simulink model "sampleModel2051"  (R2023a)
settings: Solver=VariableStepAuto  StartTime=0.0  StopTime=10.0  RelTol=1e-3
libraries: simulink x5, hdlsllib x4
settings Model: Creator=user1  LastModifiedBy=user1

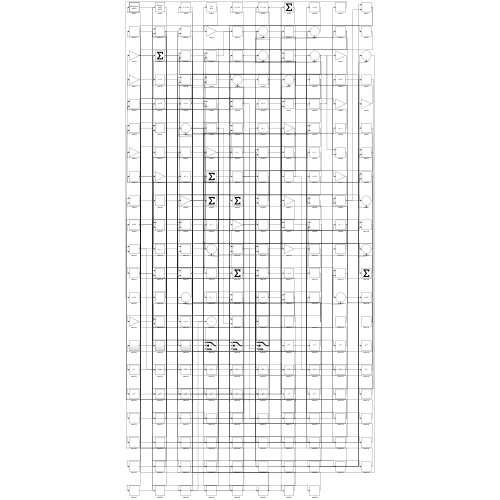
[thumbnail: Simulink's stored preview of the top-level diagram]
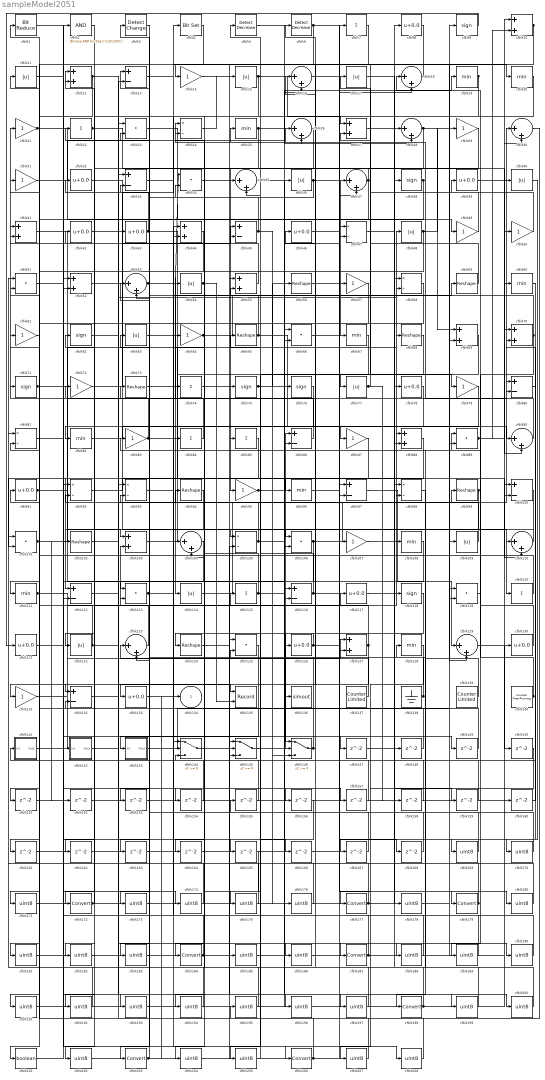
== system sampleModel2051 ==
  cfblk1 : hdlsllib/Logic and Bit Operations/Bit Reduce  mode=AND
  cfblk{10,12,27,41,44,52,55,69..70,88,103,127} (12 alike) : Sum
  cfblk{13,33,45,80,86,97,100,112,116,132} (10 alike) : Sum  Inputs=+-
  cfblk{23,34,51,66,89,101,106,113,119,125} (10 alike) : DotProduct  OutDataTypeStr=Inherit: Inherit via internal rule
  cfblk{56,59,65,68,73,94,99,102,124} (9 alike) : Reshape
  cfblk{16,18,26,28,30,35,37,53,90,104,110,123,129} (13 alike) : Sum  Inputs=|++
  cfblk{24,47,58,81,92..93,98,105} (8 alike) : Product  Inputs=*/  RndMeth=Zero  SaturateOnIntegerOverflow=on
  cfblk{14,21,29,31,49..50,57,61,64,72,79,83,87,95,107,131} (16 alike) : Gain
  cfblk{19..20,25,60,67,82,96,108,111,128} (10 alike) : MinMax
  cfblk{11,15,17,36,40,48,54,63,77,109,114,122} (12 alike) : Abs  SaturateOnIntegerOverflow=off
  cfblk{7,22,74,84..85,115,120} (7 alike) : Sum  Inputs=+
  cfblk{8,32,39,42..43,46,78,91,117,121,126,130,133} (13 alike) : Bias  Bias=0.0  SaturateOnIntegerOverflow=off
  cfblk{9,38,62,71,75..76,118} (7 alike) : Signum
  cfblk135 : Record  FileSettingsInternal="{\"entries\":[{\"content\":{\"excelSettings\":{\"content\":{},\"type\":\"Streamout.ExcelSettings\"}},\"type\":\"Streamout.FileSettingStorage\",\"uuid\":\"\"}],\"packageUris\":[\"http:\\/\\/schema.mathworks.com\\/mf0\\/streamout_blocks\\/R2020a\"],\"version\":\"1.0\"}"  Layout=[1 1]  SignalsInternal="{\"entries\":[{\"content\":{\"signals\":[{\"content\":{\"blockPath\":[],\"dimensions\":[1],\"domain\":\"\",\"lineColor\":\"#a2142f\",\"plots\":[1],\"port\":1,\"signalID\":6285,\"signalName\":\"XY Graph:1\"},\"type\":\"RecordBlkView.Signal\",\"uuid\":\"\"},{\"content\":{\"blockPath\":[],\"dimensions\":[1],\"domain\":\"\",\"lineColor\":\"#139fff\",\"plots\":[1],\"port\":2,\"signalID\":6288,\"signalName\":\"XY Graph:2\"},\"type\":\"RecordBlkView.Signal\",\"uuid\":\"\"}]},\"type\":\"RecordBlkView.InputSignals\",\"uuid\":\"\"}],\"packageUris\":[\"http:\\/\\/schema.mathworks.com\\/mf0\\/streamout_blocks\\/R2020a\"],\"version\":\"1.0\"}"  VisualizationBindings="{\"xyplotplugin\":{\"info\":[{\"series\":[{\"bindingParametersList\":[{\"parameter\":\"X-Axis\",\"signalID\":6285,\"signalName\":\"XY Graph:1\"},{\"parameter\":\"Y-Axis\",\"signalID\":6288,\"signalName\":\"XY Graph:2\"}],\"seriesID\":30765}],\"subplotID\":1}]}}"  CompatibilityTag=XY  st=-1
  cfblk136 : ToWorkspace  VariableName=simout  SaveFormat=Timeseries  SampleTime=-1
  cfblk137 : hdlsllib/Sources/Counter Limited  uplimit=7  tsamp=-1
  cfblk138 : Ground
  cfblk139 : hdlsllib/Sources/Counter Limited  uplimit=7  tsamp=-1
  cfblk140 : hdlsllib/Sources/Counter Free-Running  NumBits=16  tsamp=-1
  cfblk141 : Subsystem
      settings: LibrarySourceBlock=|
      | hdlsllib/Ports &
      | Subsystems/Subsystem
  cfblk142 : Subsystem
      settings: LibrarySourceBlock=|
      | hdlsllib/Ports &
      | Subsystems/Subsystem
  cfblk143 : Subsystem
      settings: LibrarySourceBlock=|
      | hdlsllib/Ports &
      | Subsystems/Subsystem
  cfblk144 : Switch  SaturateOnIntegerOverflow=off  InputSameDT=off
  cfblk145 : Switch  SaturateOnIntegerOverflow=off  InputSameDT=off
  cfblk146 : Switch  SaturateOnIntegerOverflow=off  InputSameDT=off
  cfblk{147..168} (22 alike) : Delay  SampleTime=1
  cfblk{169..171,173..176,178,180..183,185..186,188..197,199..200,202,204..205,207..208} (31 alike) : DataTypeConversion  OutDataTypeStr=uint8  SaturateOnIntegerOverflow=off  RndMeth=Floor
  cfblk{172,177,179,184,187,198,203,206} (8 alike) : DataTypeConversion  SaturateOnIntegerOverflow=off  RndMeth=Floor
  cfblk2 : simulink/Logic and Bit Operations/Bitwise Operator  logicop=AND  UseBitMask=on  BitMask=bin2dec('11011001')  BitMaskRealWorld=Stored Integer
      settings: LibrarySourceBlock=|
      | hdlsllib/Logic and Bit
      | Operations/Bitwise
      | Operator
  cfblk201 : DataTypeConversion  OutDataTypeStr=boolean  SaturateOnIntegerOverflow=off  RndMeth=Floor
  cfblk3 : simulink/Logic and Bit Operations/Detect Change  vinit=0  OutDataTypeStr=boolean
      settings: LibrarySourceBlock=|
      | hdlsllib/Logic and Bit
      | Operations/Detect
      | Change
  cfblk4 : simulink/Logic and Bit Operations/Bit Set  iBit=0
      settings: LibrarySourceBlock=|
      | hdlsllib/Logic and Bit
      | Operations/Bit Set
  cfblk5 : simulink/Logic and Bit Operations/Detect Decrease  vinit=0.0  OutDataTypeStr=boolean
      settings: LibrarySourceBlock=|
      | hdlsllib/Logic and Bit
      | Operations/Detect
      | Decrease
  cfblk6 : simulink/Logic and Bit Operations/Detect Decrease  vinit=0.0  OutDataTypeStr=boolean
      settings: LibrarySourceBlock=|
      | hdlsllib/Logic and Bit
      | Operations/Detect
      | Decrease
  cfblk134 : Outport  VectorParamsAs1DForOutWhenUnconnected=off
  wires:
  cfblk48/1 -> cfblk114/1, cfblk29/1
  cfblk41/1 -> cfblk103/1
  cfblk141/1(Out1) -> cfblk127/1
  cfblk145/1 -> cfblk86/1
  cfblk18/1 -> cfblk14/1
  cfblk66/1 -> cfblk37/1
  cfblk64/1 -> cfblk38/1, cfblk204/1
  cfblk55/1 -> cfblk42/1
  cfblk88/1 -> cfblk112/1
  cfblk78/1 -> cfblk172/1
  cfblk3/1 -> cfblk143/1(In1)
  cfblk84/1 -> cfblk21/1
  cfblk90/1 -> cfblk26/1
  cfblk9/1 -> cfblk121/1
  cfblk26/1 -> cfblk95/1
  cfblk60/1 -> cfblk141/1(In1)
  cfblk72/1 -> cfblk45/1
  cfblk117/1 -> cfblk48/1
  cfblk10/1 -> cfblk77/1, cfblk69/2
  cfblk146/1 -> cfblk46/1, cfblk92/2
  cfblk23/1 -> cfblk49/1
  cfblk111/1 -> cfblk117/1, cfblk145/2
  cfblk15/1 -> cfblk27/1, cfblk44/2
  cfblk103/1 -> cfblk68/1
  cfblk125/1 -> cfblk203/1
  cfblk32/1 -> cfblk120/1
  cfblk140/1 -> cfblk18/1, cfblk83/1
  cfblk118/1 -> cfblk146/1
  cfblk112/1 -> cfblk33/1
  cfblk92/1 -> cfblk96/1
  cfblk21/1 -> cfblk55/1, cfblk166/1
  cfblk47/1 -> cfblk28/1
  cfblk65/1 -> cfblk87/1, cfblk23/2
  cfblk8/1 -> cfblk136/1
  cfblk59/1 -> cfblk27/2
  cfblk126/1 -> cfblk118/1, cfblk124/1
  cfblk123/1 -> cfblk103/2
  cfblk143/1(Out1) -> cfblk9/1
  cfblk113/1 -> cfblk59/1, cfblk173/1
  cfblk114/1 -> cfblk30/1
  cfblk25/1 -> cfblk28/2, cfblk82/1
  cfblk105/1 -> cfblk13/1, cfblk146/3, cfblk197/1
  cfblk53/1 -> cfblk34/1, cfblk156/1, cfblk157/1
  cfblk70/1 -> cfblk22/1, cfblk189/1
  cfblk49/1 -> cfblk24/1
  cfblk97/1 -> cfblk129/1
  cfblk69/1 -> cfblk86/2
  cfblk35/1 -> cfblk76/1
  cfblk37/1 -> cfblk35/1, cfblk201/1
  cfblk137/1 -> cfblk123/1
  cfblk115/1 -> cfblk41/1, cfblk199/1
  cfblk100/1 -> cfblk184/1
  cfblk128/1 -> cfblk177/1
  cfblk91/1 -> cfblk8/1, cfblk154/1
  cfblk77/1 -> cfblk17/1, cfblk158/1
  cfblk13/1 -> cfblk20/1
  cfblk31/1 -> cfblk19/1
  cfblk87/1 -> cfblk101/2
  cfblk127/1 -> cfblk12/1, cfblk151/1, cfblk163/1
  cfblk46/1 -> cfblk97/1
  cfblk24/1 -> cfblk15/1
  cfblk138/1 -> cfblk73/1, cfblk127/2, cfblk41/2
  cfblk144/1 -> cfblk187/1
  cfblk45/1 -> cfblk3/1, cfblk176/1
  cfblk89/1 -> cfblk10/1, cfblk10/2
  cfblk139/1 -> cfblk88/1
  cfblk28/1 -> cfblk123/2, cfblk88/2, cfblk69/1
  cfblk116/1 -> cfblk7/1, cfblk5/1
  cfblk73/1 -> cfblk90/1
  cfblk109/1 -> cfblk94/1
  cfblk43/1 -> cfblk145/1, cfblk32/1
  cfblk11/1 -> cfblk142/1(In1)
  cfblk36/1 -> cfblk34/2, cfblk89/2
  cfblk58/1 -> cfblk75/1
  cfblk50/1 -> cfblk25/1
  cfblk110/1 -> cfblk105/1
  cfblk12/1 -> cfblk161/1, cfblk162/1, cfblk200/1
  cfblk14/1 -> cfblk97/2
  cfblk101/1 -> cfblk80/1, cfblk152/1
  cfblk29/1 -> cfblk133/1
  cfblk104/1 -> cfblk112/2
  cfblk122/1 -> cfblk99/1, cfblk11/1
  cfblk120/1 -> cfblk91/1
  cfblk98/1 -> cfblk198/1
  cfblk54/1 -> cfblk104/1, cfblk135/2
  cfblk95/1 -> cfblk47/1, cfblk149/1
  cfblk96/1 -> cfblk18/2
  cfblk75/1 -> cfblk110/1, cfblk56/1, cfblk190/1
  cfblk7/1 -> cfblk45/2
  cfblk52/1 -> cfblk4/1
  cfblk39/1 -> cfblk90/2
  cfblk5/1 -> cfblk26/2
  cfblk19/1 -> cfblk113/1, cfblk104/2
  cfblk83/1 -> cfblk110/2, cfblk80/2, cfblk31/1, cfblk106/2
  cfblk68/1 -> cfblk106/1
  cfblk71/1 -> cfblk52/2, cfblk126/1
  cfblk44/1 -> cfblk111/1
  cfblk63/1 -> cfblk79/1
  cfblk16/1 -> cfblk179/1
  cfblk99/1 -> cfblk39/1, cfblk192/1
  cfblk22/1 -> cfblk129/2, cfblk60/1
  cfblk93/1 -> cfblk206/1
  cfblk82/1 -> cfblk84/1
  cfblk86/1 -> cfblk54/1
  cfblk133/1 -> cfblk55/2
  cfblk106/1 -> cfblk70/1, cfblk164/1
  cfblk62/1 -> cfblk135/1
  cfblk131/1 -> cfblk43/1
  cfblk76/1 -> cfblk132/1
  cfblk33/1 -> cfblk85/1
  cfblk79/1 -> cfblk146/2
  cfblk142/1(Out1) -> cfblk115/1
  cfblk132/1 -> cfblk58/2
  cfblk6/1 -> cfblk107/1, cfblk145/3
  cfblk130/1 -> cfblk89/1
  cfblk57/1 -> cfblk131/1
  cfblk38/1 -> cfblk102/1, cfblk171/1
  cfblk20/1 -> cfblk122/1
  cfblk121/1 -> cfblk147/1
  cfblk27/1 -> cfblk148/1
  cfblk148/1 -> cfblk52/1
  cfblk149/1 -> cfblk1/1
  cfblk129/1 -> cfblk150/1
  cfblk151/1 -> cfblk30/2
  cfblk152/1 -> cfblk13/2
  cfblk85/1 -> cfblk153/1
  cfblk153/1 -> cfblk33/2
  cfblk154/1 -> cfblk53/1
  cfblk155/1 -> cfblk132/2
  cfblk157/1 -> cfblk12/2
  cfblk158/1 -> cfblk35/2
  cfblk17/1 -> cfblk159/1
  cfblk159/1 -> cfblk24/2
  cfblk160/1 -> cfblk70/2
  cfblk161/1 -> cfblk105/2
  cfblk162/1 -> cfblk44/1
  cfblk163/1 -> cfblk37/2
  cfblk164/1 -> cfblk47/2
  cfblk42/1 -> cfblk165/1
  cfblk166/1 -> cfblk116/2
  cfblk40/1 -> cfblk167/1
  cfblk167/1 -> cfblk66/1
  cfblk56/1 -> cfblk168/1
  cfblk168/1 -> cfblk58/1
  cfblk119/1 -> cfblk169/1
  cfblk169/1 -> cfblk63/1
  cfblk80/1 -> cfblk170/1
  cfblk170/1 -> cfblk119/1
  cfblk171/1 -> cfblk119/2
  cfblk172/1 -> cfblk72/1, cfblk62/1
  cfblk173/1 -> cfblk78/1
  cfblk51/1 -> cfblk174/1
  cfblk174/1 -> cfblk23/1
  cfblk156/1 -> cfblk175/1
  cfblk175/1 -> cfblk51/1
  cfblk176/1 -> cfblk51/2
  cfblk177/1 -> cfblk64/1, cfblk101/1
  cfblk107/1 -> cfblk178/1
  cfblk178/1 -> cfblk128/1
  cfblk179/1 -> cfblk65/1, cfblk116/1
  cfblk147/1 -> cfblk180/1
  cfblk180/1 -> cfblk16/1
  cfblk4/1 -> cfblk181/1
  cfblk181/1 -> cfblk16/2
  cfblk108/1 -> cfblk182/1
  cfblk182/1 -> cfblk57/1
  cfblk94/1 -> cfblk183/1
  cfblk183/1 -> cfblk108/1
  cfblk184/1 -> cfblk92/1, cfblk36/1
  cfblk124/1 -> cfblk185/1
  cfblk185/1 -> cfblk100/1
  cfblk102/1 -> cfblk186/1
  cfblk186/1 -> cfblk100/2
  cfblk187/1 -> cfblk155/1, cfblk109/1
  cfblk34/1 -> cfblk188/1
  cfblk188/1 -> cfblk144/1
  cfblk189/1 -> cfblk144/2
  cfblk190/1 -> cfblk144/3
  cfblk61/1 -> cfblk191/1
  cfblk191/1 -> cfblk50/1
  cfblk192/1 -> cfblk61/1
  cfblk81/1 -> cfblk193/1
  cfblk193/1 -> cfblk66/2
  cfblk165/1 -> cfblk194/1
  cfblk194/1 -> cfblk81/1
  cfblk30/1 -> cfblk195/1
  cfblk195/1 -> cfblk81/2
  cfblk74/1 -> cfblk196/1
  cfblk196/1 -> cfblk40/1
  cfblk197/1 -> cfblk74/1
  cfblk198/1 -> cfblk160/1, cfblk130/1, cfblk6/1
  cfblk199/1 -> cfblk98/1
  cfblk200/1 -> cfblk98/2
  cfblk201/1 -> cfblk2/1
  cfblk2/1 -> cfblk202/1
  cfblk202/1 -> cfblk67/1
  cfblk203/1 -> cfblk53/2, cfblk134/1
  cfblk204/1 -> cfblk125/1
  cfblk67/1 -> cfblk205/1
  cfblk205/1 -> cfblk125/2
  cfblk206/1 -> cfblk113/2, cfblk71/1
  cfblk150/1 -> cfblk207/1
  cfblk207/1 -> cfblk93/1
  cfblk1/1 -> cfblk208/1
  cfblk208/1 -> cfblk93/2

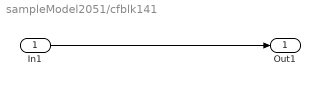
== system sampleModel2051/cfblk141 ==
  In1 : Inport
  Out1 : Outport
  wires:
  In1/1 -> Out1/1

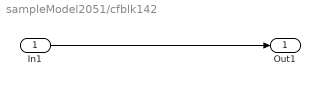
== system sampleModel2051/cfblk142 ==
  In1 : Inport
  Out1 : Outport
  wires:
  In1/1 -> Out1/1

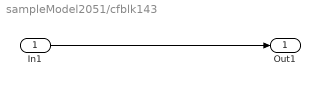
== system sampleModel2051/cfblk143 ==
  In1 : Inport
  Out1 : Outport
  wires:
  In1/1 -> Out1/1
